simulink model "modelo_SIS"  (R2019b)
settings: Solver=VariableStepAuto  StartTime=0.0  StopTime=365  RelTol=1e-3
undefined symbols (not defined in the file): beta, I0, S0
settings Model: Creator=lucia  LastModifiedBy=lucia

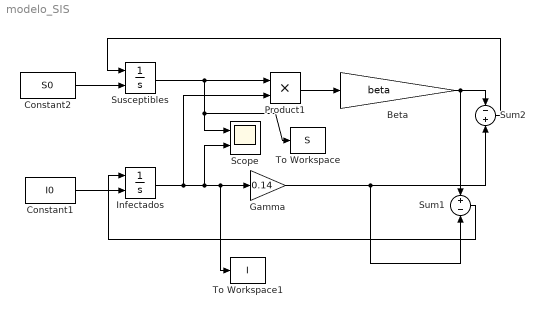
== system modelo_SIS ==
  Beta : Gain  Gain=beta
  Constant1 : Constant  Value=I0
  Constant2 : Constant  Value=S0
  Gamma : Gain  Gain=0.14
  Infectados : Integrator  InitialConditionSource=external
  Product1 : Product
  Scope : Scope  NumInputPorts=2
  Sum1 : Sum  Inputs=+-
  Sum2 : Sum  Inputs=-+
  Susceptibles : Integrator  InitialConditionSource=external
  To Workspace : ToWorkspace  VariableName=S  SaveFormat=Structure With Time  SampleTime=-1
  To Workspace1 : ToWorkspace  VariableName=I  SaveFormat=Structure With Time  SampleTime=-1
  wires:
  Constant2/1 -> Susceptibles/2
  Constant1/1 -> Infectados/2
  Susceptibles/1 -> To Workspace/1, Scope/1, Product1/1
  Infectados/1 -> Product1/2, Scope/2, To Workspace1/1, Gamma/1
  Product1/1 -> Beta/1
  Beta/1 -> Sum2/1, Sum1/1
  Sum2/1 -> Susceptibles/1
  Sum1/1 -> Infectados/1
  Gamma/1 -> Sum1/2, Sum2/2
